simulink model "filters_simulink"  (R2025b)
settings: Solver=VariableStepAuto  StartTime=0.0  StopTime=0.2  RelTol=1e-3
undefined symbols (not defined in the file or in its folder): dspblkCoreblockFVToolHelper, gcbh
libraries: simulink x2
settings Model: Creator=goma  LastModifiedBy=goma
settings SFSimCC: SimCustomHeaderCode=|
  | #include "lpf_c_caller.h"
  | #include "hpf_c_caller.h"
  | #include "apf_c_caller.h"
  | #include "bpf_c_caller.h"
  | #include "bsf_c_caller.h"
settings SFSimCC: SimUserSources=|
  | lpf_c_caller.c
  | hpf_c_caller.c
  | apf_c_caller.c
  | bpf_c_caller.c
  | bsf_c_caller.c

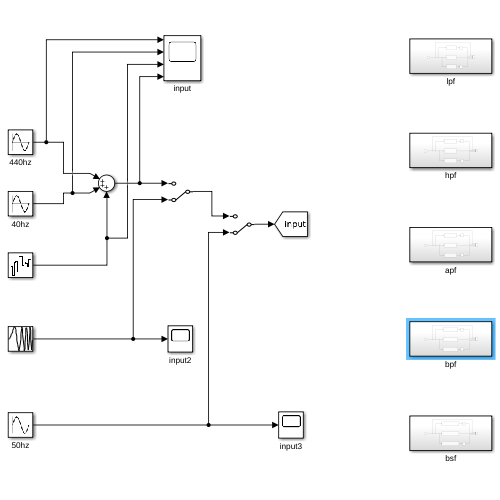
[thumbnail: Simulink's stored preview of the top-level diagram]
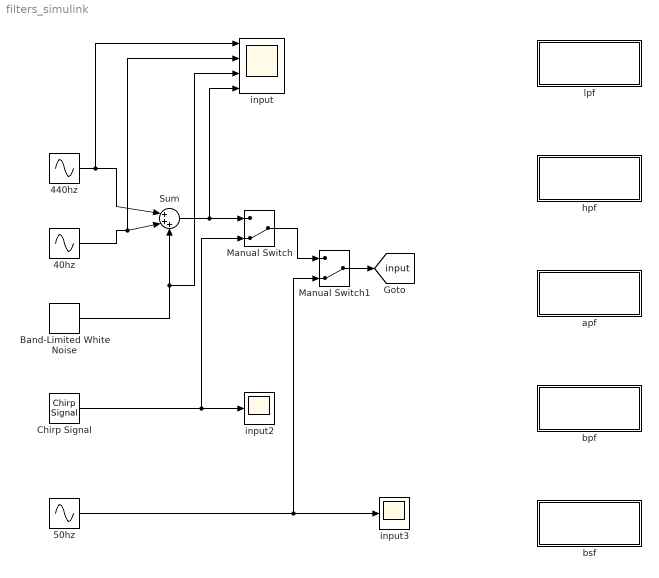
== system filters_simulink ==
  40hz : Sin  Frequency=2*pi*40  SampleTime=0
  440hz : Sin  Frequency=2*pi*440  SampleTime=0
  50hz : Sin  Frequency=2*pi*100  SampleTime=0
  Band-Limited White Noise : simulink/Sources/Band-Limited White Noise  Cov=0.05  Ts=0.0001  seed=[23341]
  Chirp Signal : simulink/Sources/Chirp Signal  f1=50  T=0.2  f2=300
  Manual Switch : ManualSwitch  CurrentSetting=0
  Manual Switch1 : ManualSwitch  CurrentSetting=0
  Sum : Sum  Inputs=|+++
  apf : Subsystem
  bpf : Subsystem
  bsf : Subsystem
  hpf : Subsystem
  input : Scope  NumInputPorts=4
  input2 : Scope
  input3 : Scope
      settings: DataLoggingVariableName=ScopeData2
  lpf : Subsystem
  tag scope: input=global
  wires:
  440hz/1 -> input/1, Sum/1
  40hz/1 -> input/2, Sum/2
  Band-Limited White Noise/1 -> input/3, Sum/3
  Sum/1 -> input/4, Manual Switch/1
  Chirp Signal/1 -> Manual Switch/2, input2/1
  50hz/1 -> input3/1, Manual Switch1/2
  Manual Switch1/1 -> [input]
  Manual Switch/1 -> Manual Switch1/1

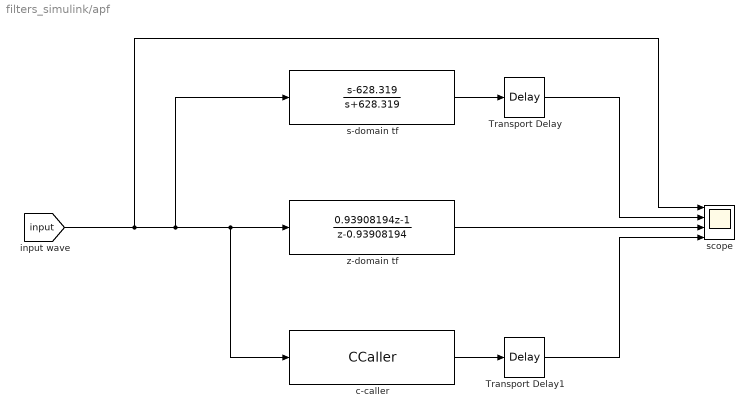
== system filters_simulink/apf ==
  Transport Delay : TransportDelay  DelayTime=0.002
  Transport Delay1 : TransportDelay  DelayTime=0.004
  c-caller : CCaller  FunctionName=apf_step  PortSpecificationStruct="%)30     .    N ,   8    (     @         %    \"     (    !     0         %  0 \"0    $    _    07)G3F%M90  4&]R=$YA;64 4V-O<&4     26YD97@     5'EP90      4VEZ90      27-';&]B86P   X    P    !@    @    $          4    (     0    ,    !         !   P!O=70 #@   #     &    \"     0         !0    @    !     P    $         $  # &]U=  .    .     8    (    !          %    \"     $    &     0         0    !@   $]U='!U=   #@   #@    &    \"     8         !0    @    !     0    $         \"0    @               X    X    !@    @    $          4    (     0    8    !         !     &    9&]U8FQE   .    ,     8    (    !          %    \"     $    !     0         0  $ ,0    X    P    !@    @    ) @        4    (     0    $    !          (  0      #@   #     &    \"     0         !0    @    !     @    $         $  \" '@P   .    ,     8    (    !          %    \"     $    \"     0         0  ( >#    X    X    !@    @    $          4    (     0    4    !         !     %    26YP=70    .    .     8    (    !@         %    \"     $    !     0         )    \"               #@   #@    &    \"     0         !0    @    !    !@    $         $     8   !D;W5B;&4   X    P    !@    @    $          4    (     0    $    !         !   0 Q    #@   #     &    \"     D\"        !0    @    !     0    $          @ !"  SampleTime=0.0001
  s-domain tf : TransferFcn  Numerator=[1 -628.319]  Denominator=[1 628.319]
  scope : Scope  NumInputPorts=4
      settings: ActiveDisplayYMinimum=-3.2010108129554125  ActiveDisplayYMaximum=1.9867147971946055  DataLoggingVariableName=ScopeData3
  z-domain tf : DiscreteTransferFcn  LoadFcn=dspblkCoreblockFVToolHelper(gcbh,'load');  Numerator=[0.93908194 -1]  Denominator=[1 -0.93908194]
      settings: CopyFcn=dspblkCoreblockFVToolHelper(gcbh,'copy');  DeleteFcn=dspblkCoreblockFVToolHelper(gcbh,'close');  ModelCloseFcn=dspblkCoreblockFVToolHelper(gcbh,'close');  PreSaveFcn=dspblkCoreblockFVToolHelper(gcbh,'presave');  PostSaveFcn=dspblkCoreblockFVToolHelper(gcbh,'postsave');  CloseFcn=dspblkCoreblockFVToolHelper(gcbh,'close');
  wires:
  s-domain tf/1 -> Transport Delay/1
  z-domain tf/1 -> scope/3
  [input] -> scope/1, c-caller/1, z-domain tf/1, s-domain tf/1
  c-caller/1 -> Transport Delay1/1
  Transport Delay/1 -> scope/2
  Transport Delay1/1 -> scope/4

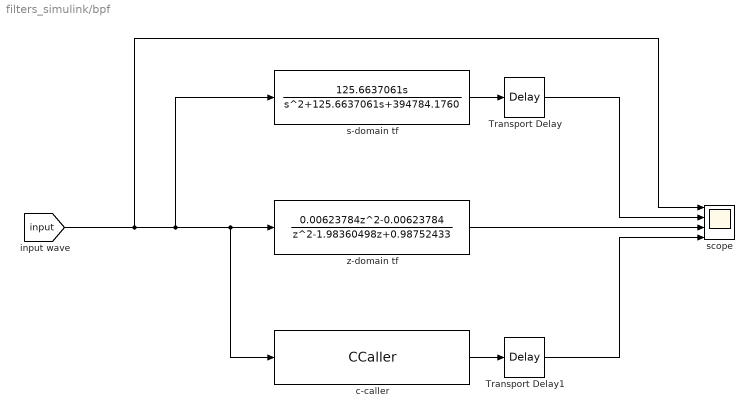
== system filters_simulink/bpf ==
  Transport Delay : TransportDelay  DelayTime=0.002
  Transport Delay1 : TransportDelay  DelayTime=0.004
  c-caller : CCaller  FunctionName=bpf_step  PortSpecificationStruct="%)30     .    N ,   8    (     @         %    \"     (    !     0         %  0 \"0    $    _    07)G3F%M90  4&]R=$YA;64 4V-O<&4     26YD97@     5'EP90      4VEZ90      27-';&]B86P   X    P    !@    @    $          4    (     0    ,    !         !   P!O=70 #@   #     &    \"     0         !0    @    !     P    $         $  # &]U=  .    .     8    (    !          %    \"     $    &     0         0    !@   $]U='!U=   #@   #@    &    \"     8         !0    @    !     0    $         \"0    @               X    X    !@    @    $          4    (     0    8    !         !     &    9&]U8FQE   .    ,     8    (    !          %    \"     $    !     0         0  $ ,0    X    P    !@    @    ) @        4    (     0    $    !          (  0      #@   #     &    \"     0         !0    @    !     @    $         $  \" '@P   .    ,     8    (    !          %    \"     $    \"     0         0  ( >#    X    X    !@    @    $          4    (     0    4    !         !     %    26YP=70    .    .     8    (    !@         %    \"     $    !     0         )    \"               #@   #@    &    \"     0         !0    @    !    !@    $         $     8   !D;W5B;&4   X    P    !@    @    $          4    (     0    $    !         !   0 Q    #@   #     &    \"     D\"        !0    @    !     0    $          @ !"  SampleTime=0.0001
  s-domain tf : TransferFcn  Numerator=[0 125.6637061 0]  Denominator=[1 125.6637061 394784.1760]
  scope : Scope  NumInputPorts=4
      settings: ActiveDisplayYMinimum=-3.2010108129554125  ActiveDisplayYMaximum=1.9867147971946055  DataLoggingVariableName=ScopeData3
  z-domain tf : DiscreteTransferFcn  LoadFcn=dspblkCoreblockFVToolHelper(gcbh,'load');  Numerator=[0.00623784 0 -0.00623784]  Denominator=[1 -1.98360498 0.98752433]
      settings: CopyFcn=dspblkCoreblockFVToolHelper(gcbh,'copy');  DeleteFcn=dspblkCoreblockFVToolHelper(gcbh,'close');  ModelCloseFcn=dspblkCoreblockFVToolHelper(gcbh,'close');  PreSaveFcn=dspblkCoreblockFVToolHelper(gcbh,'presave');  PostSaveFcn=dspblkCoreblockFVToolHelper(gcbh,'postsave');  CloseFcn=dspblkCoreblockFVToolHelper(gcbh,'close');
  wires:
  s-domain tf/1 -> Transport Delay/1
  z-domain tf/1 -> scope/3
  [input] -> scope/1, c-caller/1, z-domain tf/1, s-domain tf/1
  c-caller/1 -> Transport Delay1/1
  Transport Delay/1 -> scope/2
  Transport Delay1/1 -> scope/4

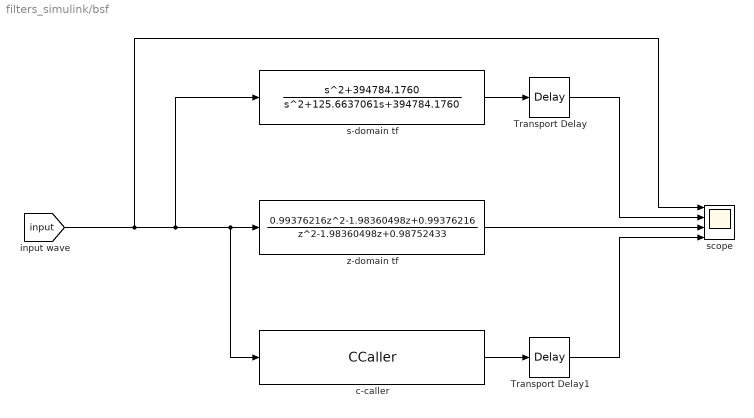
== system filters_simulink/bsf ==
  Transport Delay : TransportDelay  DelayTime=0.002
  Transport Delay1 : TransportDelay  DelayTime=0.004
  c-caller : CCaller  FunctionName=bsf_step  PortSpecificationStruct="%)30     .    N ,   8    (     @         %    \"     (    !     0         %  0 \"0    $    _    07)G3F%M90  4&]R=$YA;64 4V-O<&4     26YD97@     5'EP90      4VEZ90      27-';&]B86P   X    P    !@    @    $          4    (     0    ,    !         !   P!O=70 #@   #     &    \"     0         !0    @    !     P    $         $  # &]U=  .    .     8    (    !          %    \"     $    &     0         0    !@   $]U='!U=   #@   #@    &    \"     8         !0    @    !     0    $         \"0    @               X    X    !@    @    $          4    (     0    8    !         !     &    9&]U8FQE   .    ,     8    (    !          %    \"     $    !     0         0  $ ,0    X    P    !@    @    ) @        4    (     0    $    !          (  0      #@   #     &    \"     0         !0    @    !     @    $         $  \" '@P   .    ,     8    (    !          %    \"     $    \"     0         0  ( >#    X    X    !@    @    $          4    (     0    4    !         !     %    26YP=70    .    .     8    (    !@         %    \"     $    !     0         )    \"               #@   #@    &    \"     0         !0    @    !    !@    $         $     8   !D;W5B;&4   X    P    !@    @    $          4    (     0    $    !         !   0 Q    #@   #     &    \"     D\"        !0    @    !     0    $          @ !"  SampleTime=0.0001
  s-domain tf : TransferFcn  Numerator=[1 0 394784.1760]  Denominator=[1 125.6637061 394784.1760]
  scope : Scope  NumInputPorts=4
      settings: ActiveDisplayYMinimum=-3.2010108129554125  ActiveDisplayYMaximum=1.9867147971946055  YLabel=amplitud  DataLoggingVariableName=ScopeData3
  z-domain tf : DiscreteTransferFcn  LoadFcn=dspblkCoreblockFVToolHelper(gcbh,'load');  Numerator=[0.99376216 -1.98360498 0.99376216]  Denominator=[1 -1.98360498 0.98752433]
      settings: CopyFcn=dspblkCoreblockFVToolHelper(gcbh,'copy');  DeleteFcn=dspblkCoreblockFVToolHelper(gcbh,'close');  ModelCloseFcn=dspblkCoreblockFVToolHelper(gcbh,'close');  PreSaveFcn=dspblkCoreblockFVToolHelper(gcbh,'presave');  PostSaveFcn=dspblkCoreblockFVToolHelper(gcbh,'postsave');  CloseFcn=dspblkCoreblockFVToolHelper(gcbh,'close');
  wires:
  s-domain tf/1 -> Transport Delay/1
  z-domain tf/1 -> scope/3
  [input] -> scope/1, c-caller/1, z-domain tf/1, s-domain tf/1
  c-caller/1 -> Transport Delay1/1
  Transport Delay/1 -> scope/2
  Transport Delay1/1 -> scope/4

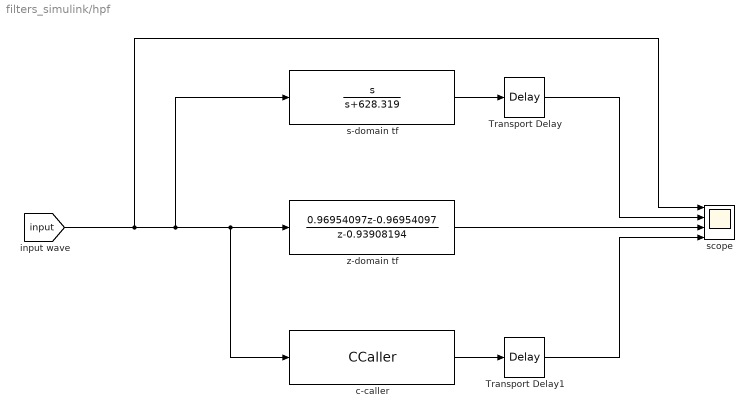
== system filters_simulink/hpf ==
  Transport Delay : TransportDelay  DelayTime=0.002
  Transport Delay1 : TransportDelay  DelayTime=0.004
  c-caller : CCaller  FunctionName=hpf_step  PortSpecificationStruct="%)30     .    N ,   8    (     @         %    \"     (    !     0         %  0 \"0    $    _    07)G3F%M90  4&]R=$YA;64 4V-O<&4     26YD97@     5'EP90      4VEZ90      27-';&]B86P   X    P    !@    @    $          4    (     0    ,    !         !   P!O=70 #@   #     &    \"     0         !0    @    !     P    $         $  # &]U=  .    .     8    (    !          %    \"     $    &     0         0    !@   $]U='!U=   #@   #@    &    \"     8         !0    @    !     0    $         \"0    @               X    X    !@    @    $          4    (     0    8    !         !     &    9&]U8FQE   .    ,     8    (    !          %    \"     $    !     0         0  $ ,0    X    P    !@    @    ) @        4    (     0    $    !          (  0      #@   #     &    \"     0         !0    @    !     @    $         $  \" '@P   .    ,     8    (    !          %    \"     $    \"     0         0  ( >#    X    X    !@    @    $          4    (     0    4    !         !     %    26YP=70    .    .     8    (    !@         %    \"     $    !     0         )    \"               #@   #@    &    \"     0         !0    @    !    !@    $         $     8   !D;W5B;&4   X    P    !@    @    $          4    (     0    $    !         !   0 Q    #@   #     &    \"     D\"        !0    @    !     0    $          @ !"  SampleTime=0.0001
  s-domain tf : TransferFcn  Numerator=[1 0]  Denominator=[1 628.319]
  scope : Scope  NumInputPorts=4
      settings: ActiveDisplayYMinimum=-3.2474138199887865  ActiveDisplayYMaximum=1.9981075354731477  DataLoggingVariableName=ScopeData3
  z-domain tf : DiscreteTransferFcn  LoadFcn=dspblkCoreblockFVToolHelper(gcbh,'load');  Numerator=[0.96954097 -0.96954097]  Denominator=[1 -0.93908194]
      settings: CopyFcn=dspblkCoreblockFVToolHelper(gcbh,'copy');  DeleteFcn=dspblkCoreblockFVToolHelper(gcbh,'close');  ModelCloseFcn=dspblkCoreblockFVToolHelper(gcbh,'close');  PreSaveFcn=dspblkCoreblockFVToolHelper(gcbh,'presave');  PostSaveFcn=dspblkCoreblockFVToolHelper(gcbh,'postsave');  CloseFcn=dspblkCoreblockFVToolHelper(gcbh,'close');
  wires:
  s-domain tf/1 -> Transport Delay/1
  z-domain tf/1 -> scope/3
  [input] -> scope/1, c-caller/1, z-domain tf/1, s-domain tf/1
  c-caller/1 -> Transport Delay1/1
  Transport Delay/1 -> scope/2
  Transport Delay1/1 -> scope/4

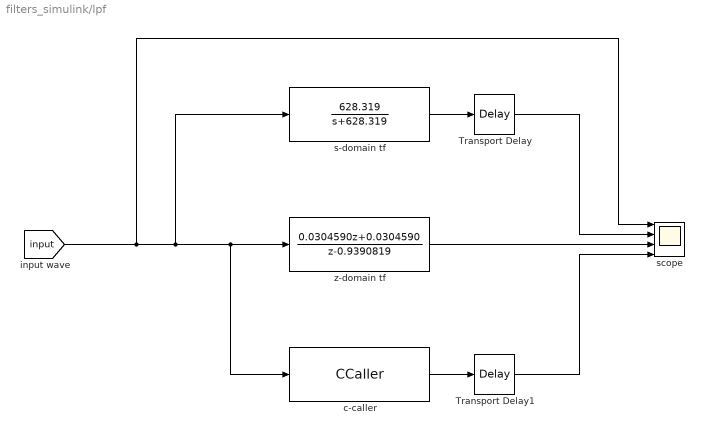
== system filters_simulink/lpf ==
  Transport Delay : TransportDelay  DelayTime=0.002
  Transport Delay1 : TransportDelay  DelayTime=0.004
  c-caller : CCaller  FunctionName=lpf_step  PortSpecificationStruct="%)30     .    N ,   8    (     @         %    \"     (    !     0         %  0 \"0    $    _    07)G3F%M90  4&]R=$YA;64 4V-O<&4     26YD97@     5'EP90      4VEZ90      27-';&]B86P   X    P    !@    @    $          4    (     0    ,    !         !   P!O=70 #@   #     &    \"     0         !0    @    !     P    $         $  # &]U=  .    .     8    (    !          %    \"     $    &     0         0    !@   $]U='!U=   #@   #@    &    \"     8         !0    @    !     0    $         \"0    @               X    X    !@    @    $          4    (     0    8    !         !     &    9&]U8FQE   .    ,     8    (    !          %    \"     $    !     0         0  $ ,0    X    P    !@    @    ) @        4    (     0    $    !          (  0      #@   #     &    \"     0         !0    @    !     @    $         $  \" '@P   .    ,     8    (    !          %    \"     $    \"     0         0  ( >#    X    X    !@    @    $          4    (     0    4    !         !     %    26YP=70    .    .     8    (    !@         %    \"     $    !     0         )    \"               #@   #@    &    \"     0         !0    @    !    !@    $         $     8   !D;W5B;&4   X    P    !@    @    $          4    (     0    $    !         !   0 Q    #@   #     &    \"     D\"        !0    @    !     0    $          @ !"  SampleTime=0.0001
  s-domain tf : TransferFcn  Numerator=[628.319]  Denominator=[1 628.319]
  scope : Scope  NumInputPorts=4
      settings: ActiveDisplayYMinimum=-1.0370380681704505  ActiveDisplayYMaximum=1.1998156172727978  DataLoggingVariableName=ScopeData3
  z-domain tf : DiscreteTransferFcn  LoadFcn=dspblkCoreblockFVToolHelper(gcbh,'load');  Numerator=[0.0304590 0.0304590]  Denominator=[1 -0.9390819]
      settings: CopyFcn=dspblkCoreblockFVToolHelper(gcbh,'copy');  DeleteFcn=dspblkCoreblockFVToolHelper(gcbh,'close');  ModelCloseFcn=dspblkCoreblockFVToolHelper(gcbh,'close');  PreSaveFcn=dspblkCoreblockFVToolHelper(gcbh,'presave');  PostSaveFcn=dspblkCoreblockFVToolHelper(gcbh,'postsave');  CloseFcn=dspblkCoreblockFVToolHelper(gcbh,'close');
  wires:
  s-domain tf/1 -> Transport Delay/1
  z-domain tf/1 -> scope/3
  [input] -> scope/1, c-caller/1, z-domain tf/1, s-domain tf/1
  c-caller/1 -> Transport Delay1/1
  Transport Delay/1 -> scope/2
  Transport Delay1/1 -> scope/4
